simulink model "sampleModel1959_5_sub"  (R2023a)
settings: Solver=VariableStepAuto  StartTime=0.0  StopTime=10.0  RelTol=1e-3
libraries: hdlsllib x3, simulink x1
settings Model: Creator=user1  LastModifiedBy=user1
settings OptimizationCC: BlockReduction=off  ConditionallyExecuteInputs=off

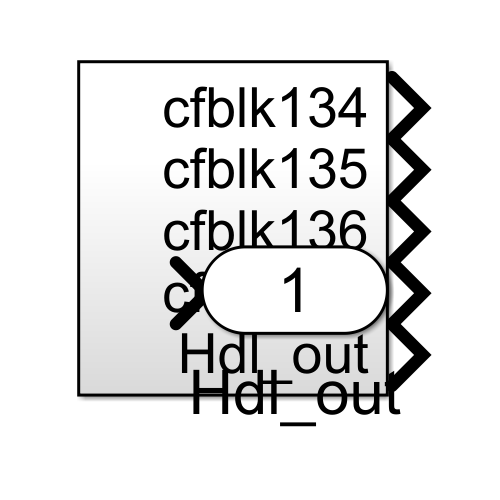
[thumbnail: Simulink's stored preview of the top-level diagram]
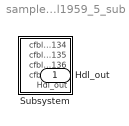
== system sampleModel1959_5_sub ==
  Subsystem : Subsystem
  Hdl_out : Outport  OutDataTypeStr=uint8

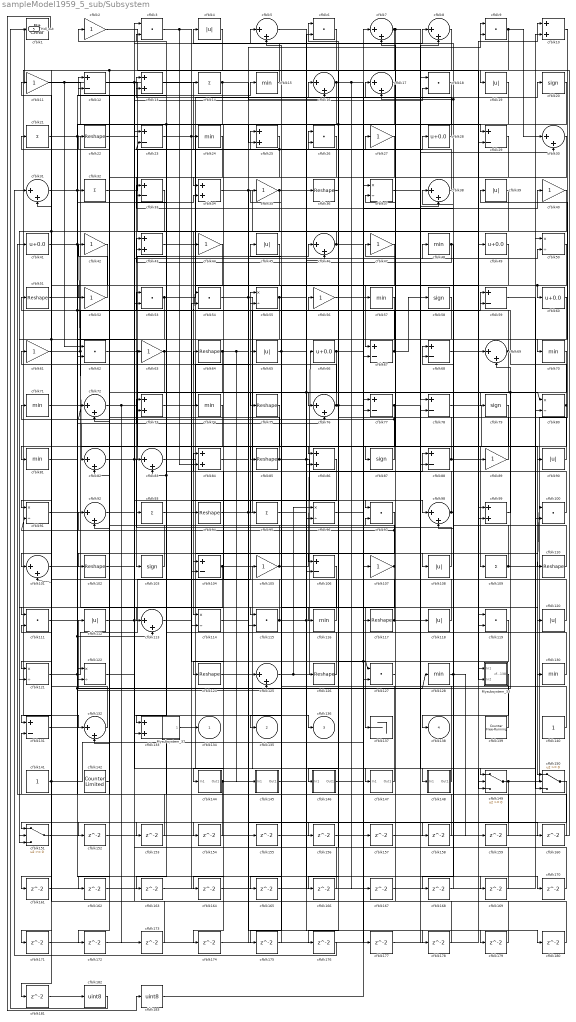
== system sampleModel1959_5_sub/Subsystem ==
  Mysubsystem_33 : Subsystem  TreatAsAtomicUnit=on  RTWFcnName=Mysubsystem_33
      settings: RTWFcnNameOpts=User specified  RTWFileNameOpts=Use function name
  Mysubsystem_37 : Subsystem  TreatAsAtomicUnit=on  RTWFcnName=Mysubsystem_37
      settings: RTWFcnNameOpts=User specified  RTWFileNameOpts=Use function name
  cfblk1 : simulink/Logic and Bit Operations/Bit Clear  iBit=0
      settings: LibrarySourceBlock=|
      | hdlsllib/Logic and Bit
      | Operations/Bit Clear
  cfblk{10,13,25,34,43,73,84,86,99,133} (10 alike) : Sum  OutDataTypeStr=uint8
  cfblk{3,6,9,18,26,53..54,62,97,100,111,115,119,127} (14 alike) : DotProduct  OutDataTypeStr=uint8
  cfblk{5,7..8,16..17,30..31,38,46,69,72,76,82..83,92,98,101,113,125,132} (20 alike) : Sum  Inputs=|++  OutDataTypeStr=uint8
  cfblk{22,36,51,64,75,85,94,102,110,117,124,126} (12 alike) : Reshape
  cfblk{20,58,79,87,103} (5 alike) : Signum
  cfblk{12,23,29,33,59,67..68,77..78,88,104,106,131} (13 alike) : Sum  Inputs=+-  OutDataTypeStr=uint8
  cfblk{2,11,27,35,40,42,44,47,52,56,61,63,89,105,107} (15 alike) : Gain  OutDataTypeStr=uint8
  cfblk{4,19,39,45,65,90,108,112,118,120} (10 alike) : Abs  OutDataTypeStr=uint8  SaturateOnIntegerOverflow=off
  cfblk{14,21,32,93,95,109} (6 alike) : Sum  Inputs=+  OutDataTypeStr=uint8
  cfblk{37,50,55,80,91,96,114,121..122} (9 alike) : Product  Inputs=*/  OutDataTypeStr=uint8  RndMeth=Zero  SaturateOnIntegerOverflow=on
  cfblk{15,24,48,57,70..71,74,81,116,128,130} (11 alike) : MinMax  OutDataTypeStr=uint8
  cfblk137 : Terminator
  cfblk139 : hdlsllib/Sources/Counter Free-Running  NumBits=16  tsamp=-1
  cfblk140 : Constant  OutDataTypeStr=uint8  SampleTime=-1
  cfblk141 : Constant  OutDataTypeStr=uint8  SampleTime=-1
  cfblk142 : hdlsllib/Sources/Counter Limited  uplimit=7  tsamp=-1
  cfblk144 : Subsystem
      settings: LibrarySourceBlock=|
      | hdlsllib/Ports &
      | Subsystems/Subsystem
  cfblk145 : Subsystem
      settings: LibrarySourceBlock=|
      | hdlsllib/Ports &
      | Subsystems/Subsystem
  cfblk146 : Subsystem
      settings: LibrarySourceBlock=|
      | hdlsllib/Ports &
      | Subsystems/Subsystem
  cfblk147 : Subsystem
      settings: LibrarySourceBlock=|
      | hdlsllib/Ports &
      | Subsystems/Subsystem
  cfblk148 : Subsystem
      settings: LibrarySourceBlock=|
      | hdlsllib/Ports &
      | Subsystems/Subsystem
  cfblk149 : Switch  OutDataTypeStr=uint8  SaturateOnIntegerOverflow=off  InputSameDT=off
  cfblk150 : Switch  OutDataTypeStr=uint8  SaturateOnIntegerOverflow=off  InputSameDT=off
  cfblk151 : Switch  OutDataTypeStr=uint8  SaturateOnIntegerOverflow=off  InputSameDT=off
  cfblk{152..181} (30 alike) : Delay  SampleTime=1
  cfblk182 : DataTypeConversion  OutDataTypeStr=uint8  SaturateOnIntegerOverflow=off  RndMeth=Floor
  cfblk183 : DataTypeConversion  OutDataTypeStr=uint8  SaturateOnIntegerOverflow=off  RndMeth=Floor
  cfblk{28,41,49,60,66} (5 alike) : Bias  Bias=0.0  SaturateOnIntegerOverflow=off
  cfblk134 : Outport  OutDataTypeStr=uint8  VectorParamsAs1DForOutWhenUnconnected=off
  cfblk135 : Outport  Port=2  OutDataTypeStr=uint8  VectorParamsAs1DForOutWhenUnconnected=off
  cfblk136 : Outport  Port=3  OutDataTypeStr=uint8  VectorParamsAs1DForOutWhenUnconnected=off
  cfblk138 : Outport  Port=4  OutDataTypeStr=uint8  VectorParamsAs1DForOutWhenUnconnected=off
  Hdl_out : Outport  Port=5  OutDataTypeStr=uint8
  wires:
  cfblk125/1 -> cfblk96/1, cfblk88/1
  cfblk53/1 -> cfblk151/1, cfblk20/1
  cfblk61/1 -> cfblk29/2, cfblk109/1
  cfblk6/1 -> cfblk132/1
  cfblk117/1 -> cfblk120/1, cfblk61/1
  cfblk70/1 -> cfblk112/1, Mysubsystem_33/2(In2)
  cfblk131/1 -> cfblk128/1, cfblk73/2, cfblk113/2
  cfblk21/1 -> cfblk29/1, cfblk137/1
  cfblk149/1 -> cfblk161/1, cfblk39/1
  cfblk87/1 -> cfblk72/1, cfblk6/1
  cfblk151/1 -> cfblk19/1
  cfblk31/1 -> cfblk63/1, cfblk32/1
  cfblk24/1 -> cfblk103/1
  cfblk121/1 -> cfblk76/2, cfblk55/1
  cfblk41/1 -> cfblk169/1, cfblk82/1
  cfblk50/1 -> cfblk53/2, cfblk60/1
  cfblk42/1 -> cfblk111/1
  cfblk85/1 -> cfblk21/1, cfblk178/1, cfblk98/1
  cfblk16/1 -> cfblk113/1, cfblk167/1, cfblk149/3
  cfblk63/1 -> cfblk82/2, cfblk127/2, cfblk127/1
  cfblk23/1 -> cfblk115/2, cfblk148/1(In1)
  cfblk105/1 -> cfblk53/1, cfblk66/1
  cfblk89/1 -> cfblk51/1
  cfblk39/1 -> cfblk114/1
  cfblk144/1(Out1) -> cfblk170/1, cfblk41/1
  cfblk104/1 -> cfblk151/2, cfblk149/1
  cfblk141/1 -> cfblk101/2, cfblk77/1
  cfblk33/1 -> cfblk131/1
  cfblk28/1 -> cfblk13/1
  cfblk67/1 -> cfblk35/1, cfblk58/1
  cfblk81/1 -> cfblk34/2, cfblk54/1
  cfblk133/1 -> cfblk43/1
  cfblk82/1 -> cfblk136/1, cfblk48/1
  cfblk108/1 -> cfblk83/1
  cfblk112/1 -> cfblk24/1, cfblk147/1(In1)
  cfblk55/1 -> cfblk28/1, cfblk104/1
  cfblk126/1 -> cfblk2/1
  cfblk113/1 -> cfblk56/1
  cfblk8/1 -> cfblk101/1
  cfblk60/1 -> cfblk86/1
  cfblk20/1 -> cfblk156/1, cfblk62/2
  cfblk64/1 -> cfblk102/1, cfblk145/1(In1), cfblk110/1
  cfblk98/1 -> cfblk168/1, cfblk16/1
  cfblk7/1 -> cfblk76/1, cfblk30/2, cfblk87/1
  cfblk62/1 -> cfblk46/1, Mysubsystem_33/1(In1)
  cfblk72/1 -> cfblk173/1, cfblk75/1
  cfblk139/1 -> cfblk25/1
  cfblk75/1 -> cfblk124/1
  cfblk93/1 -> cfblk150/1
  cfblk88/1 -> cfblk10/1, cfblk17/1
  cfblk43/1 -> cfblk89/1
  cfblk107/1 -> cfblk166/1, cfblk73/1, cfblk83/2
  cfblk120/1 -> cfblk93/1
  cfblk103/1 -> cfblk71/1
  cfblk9/1 -> cfblk30/1, cfblk106/1
  cfblk35/1 -> cfblk80/2, cfblk121/2, cfblk81/1
  cfblk36/1 -> cfblk116/1
  cfblk37/1 -> cfblk78/1
  cfblk111/1 -> cfblk15/1
  cfblk38/1 -> cfblk14/1
  cfblk128/1 -> cfblk159/1, cfblk158/1
  cfblk92/1 -> cfblk8/1
  cfblk110/1 -> cfblk17/2, cfblk4/1
  cfblk12/1 -> cfblk96/2, cfblk86/2
  cfblk99/1 -> cfblk69/2
  cfblk14/1 -> Hdl_out/1, cfblk133/1, cfblk16/2
  cfblk2/1 -> cfblk99/1
  cfblk94/1 -> cfblk180/1, cfblk9/2, cfblk59/1
  cfblk148/1(Out1) -> cfblk105/1
  cfblk78/1 -> cfblk130/1
  cfblk19/1 -> cfblk163/1, cfblk162/1
  cfblk69/1 -> cfblk3/2, cfblk135/1
  cfblk4/1 -> cfblk172/1, cfblk121/1
  cfblk97/1 -> cfblk91/2, cfblk122/2
  cfblk109/1 -> cfblk33/1, cfblk100/1
  cfblk90/1 -> cfblk68/1
  cfblk130/1 -> cfblk45/1
  cfblk100/1 -> cfblk12/1
  cfblk142/1 -> cfblk22/1
  cfblk54/1 -> cfblk79/1, cfblk97/1
  cfblk51/1 -> cfblk100/2
  cfblk3/1 -> cfblk84/2, cfblk90/1
  cfblk91/1 -> cfblk13/2
  cfblk25/1 -> cfblk153/1, cfblk23/2
  cfblk102/1 -> cfblk50/2
  cfblk140/1 -> cfblk38/1
  cfblk132/1 -> cfblk31/2
  cfblk48/1 -> cfblk43/2, cfblk98/2
  cfblk15/1 -> cfblk5/1
  cfblk95/1 -> cfblk36/1
  cfblk49/1 -> cfblk67/1
  cfblk47/1 -> cfblk95/1
  cfblk77/1 -> cfblk85/1, cfblk150/2
  cfblk32/1 -> cfblk26/1
  cfblk40/1 -> cfblk77/2
  cfblk86/1 -> cfblk114/2
  cfblk71/1 -> cfblk94/1
  cfblk18/1 -> cfblk25/2
  cfblk11/1 -> cfblk62/1, cfblk38/2
  cfblk5/1 -> cfblk126/1
  cfblk73/1 -> cfblk65/1
  cfblk116/1 -> cfblk12/2
  cfblk57/1 -> cfblk151/3, cfblk91/1
  cfblk26/1 -> cfblk52/1
  cfblk29/1 -> cfblk144/1(In1)
  cfblk127/1 -> cfblk47/1
  cfblk115/1 -> cfblk72/2, cfblk9/1, cfblk149/2
  cfblk101/1 -> cfblk125/2
  cfblk68/1 -> cfblk49/1
  cfblk22/1 -> cfblk57/1
  cfblk124/1 -> cfblk27/1
  cfblk76/1 -> cfblk11/1, cfblk40/1, cfblk146/1(In1)
  cfblk80/1 -> cfblk59/2, cfblk104/2
  cfblk10/1 -> cfblk70/1
  cfblk46/1 -> cfblk44/1, cfblk117/1
  cfblk58/1 -> cfblk74/1
  cfblk118/1 -> cfblk84/1
  cfblk65/1 -> cfblk165/1, cfblk108/1, cfblk80/1
  cfblk52/1 -> cfblk42/1
  cfblk30/1 -> cfblk34/1
  cfblk34/1 -> cfblk119/2, cfblk119/1
  cfblk13/1 -> cfblk115/1
  cfblk147/1(Out1) -> cfblk64/1
  cfblk45/1 -> cfblk92/2
  cfblk83/1 -> cfblk118/1
  cfblk56/1 -> cfblk107/1
  cfblk59/1 -> cfblk150/3
  cfblk122/1 -> cfblk18/2
  cfblk66/1 -> cfblk37/1, cfblk133/2, cfblk106/2
  cfblk74/1 -> cfblk152/1
  cfblk152/1 -> cfblk69/1
  cfblk153/1 -> cfblk132/2
  cfblk17/1 -> cfblk154/1
  cfblk154/1 -> cfblk122/1
  cfblk114/1 -> cfblk155/1
  cfblk155/1 -> cfblk6/2
  cfblk156/1 -> cfblk50/1
  cfblk96/1 -> cfblk157/1
  cfblk157/1 -> cfblk78/2
  cfblk158/1 -> cfblk92/1
  cfblk159/1 -> cfblk33/2
  cfblk84/1 -> cfblk160/1
  cfblk160/1 -> cfblk131/2
  cfblk161/1 -> cfblk10/2
  cfblk162/1 -> cfblk8/2
  cfblk163/1 -> cfblk54/2
  cfblk150/1 -> cfblk164/1
  cfblk164/1 -> cfblk67/2
  cfblk165/1 -> cfblk46/2
  cfblk166/1 -> cfblk23/1
  cfblk167/1 -> cfblk37/2
  cfblk168/1 -> cfblk68/2
  cfblk169/1 -> cfblk26/2
  cfblk170/1 -> cfblk5/2
  cfblk44/1 -> cfblk171/1
  cfblk171/1 -> cfblk125/1
  cfblk172/1 -> cfblk18/1
  cfblk173/1 -> cfblk111/2
  cfblk27/1 -> cfblk174/1
  cfblk174/1 -> cfblk99/2
  cfblk106/1 -> cfblk175/1
  cfblk175/1 -> cfblk55/2
  cfblk119/1 -> cfblk176/1
  cfblk176/1 -> cfblk31/1
  cfblk146/1(Out1) -> cfblk177/1
  cfblk177/1 -> cfblk88/2
  cfblk178/1 -> cfblk7/2
  cfblk145/1(Out1) -> cfblk179/1
  cfblk179/1 -> cfblk97/2
  cfblk180/1 -> cfblk3/1
  cfblk79/1 -> cfblk181/1
  cfblk181/1 -> cfblk182/1
  cfblk182/1 -> cfblk1/1
  cfblk1/1 -> cfblk183/1
  cfblk183/1 -> cfblk7/1
  Mysubsystem_33/1(cfblk138) -> cfblk138/1
  Mysubsystem_37/1(cfblk134) -> cfblk134/1

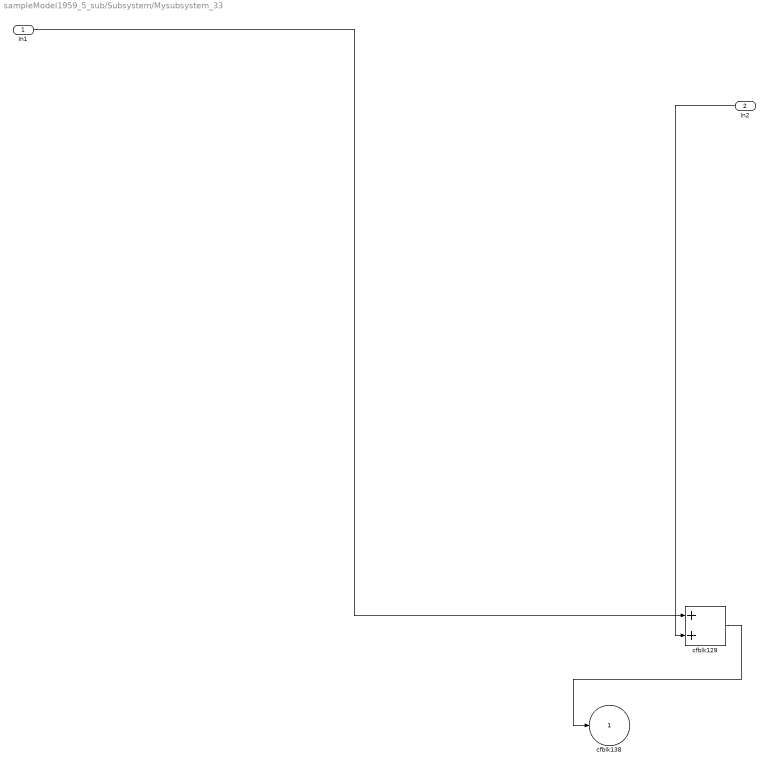
== system sampleModel1959_5_sub/Subsystem/Mysubsystem_33 ==
  In1 : Inport
  In2 : Inport  Port=2
  cfblk129 : Sum
  cfblk138 : Outport  VectorParamsAs1DForOutWhenUnconnected=off
  wires:
  In2/1 -> cfblk129/2
  cfblk129/1 -> cfblk138/1
  In1/1 -> cfblk129/1

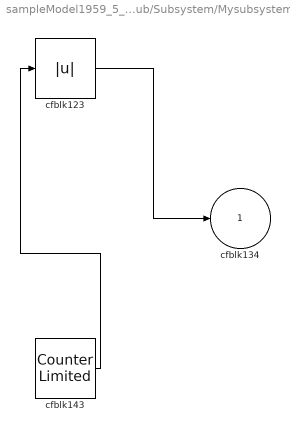
== system sampleModel1959_5_sub/Subsystem/Mysubsystem_37 ==
  cfblk123 : Abs  SaturateOnIntegerOverflow=off
  cfblk143 : hdlsllib/Sources/Counter Limited  uplimit=7  tsamp=-1
  cfblk134 : Outport  VectorParamsAs1DForOutWhenUnconnected=off
  wires:
  cfblk143/1 -> cfblk123/1
  cfblk123/1 -> cfblk134/1

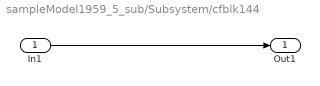
== system sampleModel1959_5_sub/Subsystem/cfblk144 ==
  In1 : Inport
  Out1 : Outport
  wires:
  In1/1 -> Out1/1

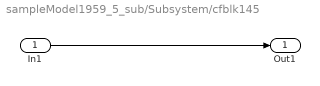
== system sampleModel1959_5_sub/Subsystem/cfblk145 ==
  In1 : Inport
  Out1 : Outport
  wires:
  In1/1 -> Out1/1

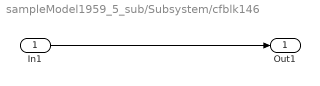
== system sampleModel1959_5_sub/Subsystem/cfblk146 ==
  In1 : Inport
  Out1 : Outport
  wires:
  In1/1 -> Out1/1

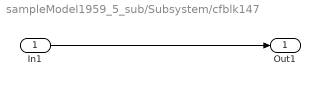
== system sampleModel1959_5_sub/Subsystem/cfblk147 ==
  In1 : Inport
  Out1 : Outport
  wires:
  In1/1 -> Out1/1

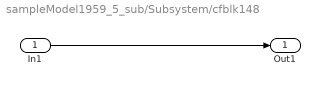
== system sampleModel1959_5_sub/Subsystem/cfblk148 ==
  In1 : Inport
  Out1 : Outport
  wires:
  In1/1 -> Out1/1
